simulink model "simu_state_space_model"  (R2015a)
settings: Solver=ode3  StartTime=0.0  StopTime=10  FixedStep=0.0001  RelTol=1e-3
values from neighbouring files (symbols this model uses):
  A = 1    [analysis_plot_decay_sin.m]
undefined symbols (not defined in the file or in its folder): B, C, D
undefined symbols (not defined in the file): A2, B2, C2, D2
settings Model: Creator=Xiaotian  LastModifiedBy=Xiaotian

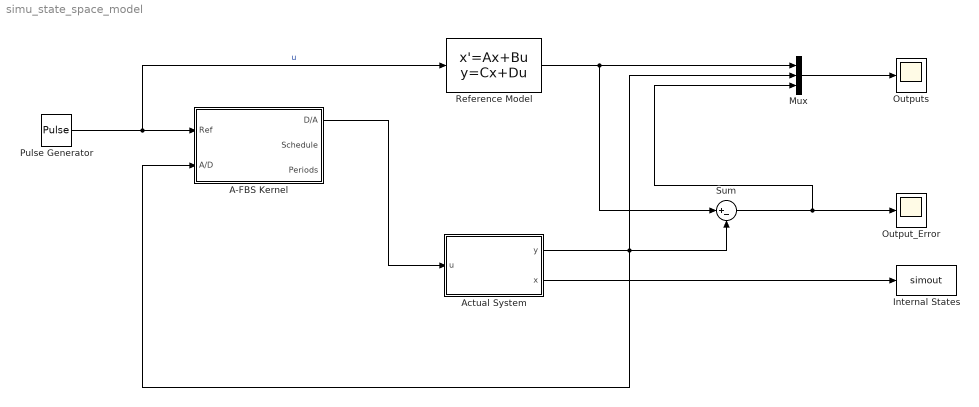
== system simu_state_space_model ==
  A-FBS Kernel : Subsystem  mask{Parameter=1}
  Actual System : Subsystem  mask{A=A2, B=B2, C=C2, D=D2}
  Internal States : ToWorkspace  VariableName=simout  SaveFormat=Timeseries  SampleTime=-1
  Mux : Mux  Inputs=3
  Output_Error : Scope
  Outputs : Scope
  Pulse Generator : DiscretePulseGenerator  PulseType=Time based  Period=30  PulseWidth=50
  Reference Model : StateSpace  A=A  B=B  C=C  D=D  X0=0
  Sum : Sum  Inputs=|+-
  wires:
  Mux/1 -> Outputs/1
  Reference Model/1 -> Sum/1, Mux/1
  Actual System/1(y) -> A-FBS Kernel/2(A/D), Mux/2, Sum/2
  Actual System/2(x) -> Internal States/1
  Sum/1 -> Mux/3, Output_Error/1
  Pulse Generator/1 -> Reference Model/1, A-FBS Kernel/1(Ref)  "u"
  A-FBS Kernel/1(D/A) -> Actual System/1(u)

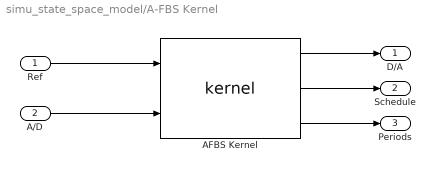
== system simu_state_space_model/A-FBS Kernel ==
  Ref : Inport
  A/D : Inport  Port=2
  AFBS Kernel : S-Function  FunctionName=kernel  Parameters=alpha, h_h, h_l
  D/A : Outport
  Schedule : Outport  Port=2
  Periods : Outport  Port=3
  wires:
  AFBS Kernel/1 -> D/A/1
  AFBS Kernel/2 -> Schedule/1
  AFBS Kernel/3 -> Periods/1
  Ref/1 -> AFBS Kernel/1
  A/D/1 -> AFBS Kernel/2

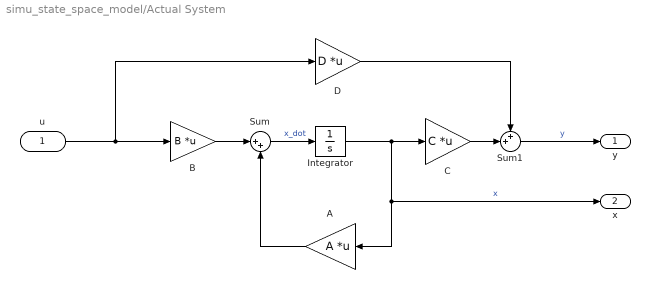
== system simu_state_space_model/Actual System ==
  u : Inport
  A : Gain  Gain=A  Multiplication=Matrix(K*u)
  B : Gain  Gain=B  Multiplication=Matrix(K*u)
  C : Gain  Gain=C  Multiplication=Matrix(K*u)
  D : Gain  Gain=D  Multiplication=Matrix(K*u)
  Integrator : Integrator
  Sum : Sum  Inputs=|++
  Sum1 : Sum  Inputs=++|
  y : Outport
  x : Outport  Port=2
  wires:
  B/1 -> Sum/1
  Sum/1 -> Integrator/1  "x_dot"
  A/1 -> Sum/2
  u/1 -> D/1, B/1
  Sum1/1 -> y/1  "y"
  D/1 -> Sum1/1
  Integrator/1 -> x/1, A/1, C/1  "x"
  C/1 -> Sum1/2
